simulink model "Q2_Simulink_Model"  (R2018a)
settings: Solver=VariableStepDiscrete  StartTime=0.0  StopTime=4  RelTol=1e-3
libraries: powerlib x22, pePowerMeasurement x4
settings Model: NumberOfSteps=10  Creator=Ataseven  LastModifiedBy=etkiacilan
settings ConfigComp: DVTestSuiteOptimization=CombinedObjectives (Nonlinear Extended)  DVDetectFloatOverflow=off

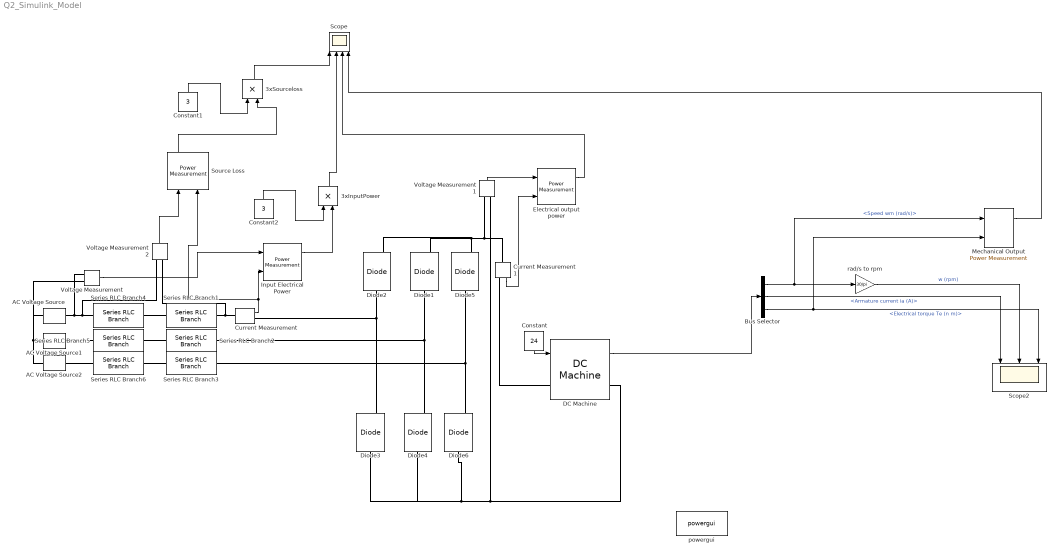
== system Q2_Simulink_Model ==
  3xInputPower : Product
  3xSourceloss : Product
  AC Voltage Source : powerlib/Electrical Sources/AC Voltage Source  Amplitude=326.59863  Phase=0  Frequency=50  SampleTime=0  Measurements=None  BusType=swing  Pref=10e3  Qref=0  Qmin=-inf  Qmax=+inf
  AC Voltage Source1 : powerlib/Electrical Sources/AC Voltage Source  Amplitude=326.59863  Phase=240  Frequency=50  SampleTime=0  Measurements=None  BusType=swing  Pref=10e3  Qref=0  Qmin=-inf  Qmax=+inf
  AC Voltage Source2 : powerlib/Electrical Sources/AC Voltage Source  Amplitude=326.59863  Phase=120  Frequency=50  SampleTime=0  Measurements=None  BusType=swing  Pref=10e3  Qref=0  Qmin=-inf  Qmax=+inf
  Bus Selector : BusSelector  OutputSignals=Speed wm (rad/s),Armature current ia (A),Electrical torque Te (n m)
  Constant : Constant  Value=24
  Constant1 : Constant  Value=3
  Constant2 : Constant  Value=3
  Current Measurement : powerlib/Measurements/Current Measurement  PhasorSimulation=off  OutputType=Complex  PSBequivalent=0
  Current Measurement1 : powerlib/Measurements/Current Measurement  PhasorSimulation=off  OutputType=Complex  PSBequivalent=0
  DC Machine : powerlib/Machines/DC Machine  PresetModel=No  MechanicalLoad=Torque TL  FieldType=Permanent magnet  ShowDetailedParameters=on  MeasurementBus=off  RLa=[ 10 0.01]  RLf="[ 240  120]"  Laf=1.8  MachineConstant=Back-emf constant (V/rpm)  Ke=0.3  Kt=1.8  J=0.4  Bm=0  Tf=0  w0=1  Ifinit=1  TsPowergui=0  TsBlock=-1
  Diode{1..6} (6 alike) : powerlib/Power Electronics/Diode  Ron=0.02  Lon=0  Vf=0.8  IC=0  UseSnubber=0  Rs=500e6  Cs=250e-9  Measurements=on
  "Electrical output power " : pePowerMeasurement/Power Measurement  OverrideUsingVariant=Discrete  F=50  K=[0 1 2 3]  Ts=10e-6
  Input Electrical Power : pePowerMeasurement/Power Measurement  OverrideUsingVariant=Discrete  F=50  K=[0 1 2 3]  Ts=10e-6
  "Mechanical Output " : pePowerMeasurement/Power Measurement  OverrideUsingVariant=Discrete  F=50  K=[0 1 2 3]  Ts=10e-6
  Scope : Scope  NumInputPorts=4
  Scope2 : Scope  NumInputPorts=3
  Series RLC Branch1 : powerlib/Elements/Series RLC Branch  LConnTagsString=__new0  RConnTagsString=__new0  BranchType=L  Resistance=1  Inductance=100e-6  SetiL0=off  InitialCurrent=0  Capacitance=1e-6  Setx0=off  InitialVoltage=0  Measurements=None
  Series RLC Branch2 : powerlib/Elements/Series RLC Branch  LConnTagsString=__new0  RConnTagsString=__new0  BranchType=L  Resistance=1  Inductance=100e-6  SetiL0=off  InitialCurrent=0  Capacitance=1e-6  Setx0=off  InitialVoltage=0  Measurements=None
  Series RLC Branch3 : powerlib/Elements/Series RLC Branch  LConnTagsString=__new0  RConnTagsString=__new0  BranchType=L  Resistance=1  Inductance=100e-6  SetiL0=off  InitialCurrent=0  Capacitance=1e-6  Setx0=off  InitialVoltage=0  Measurements=None
  Series RLC Branch4 : powerlib/Elements/Series RLC Branch  LConnTagsString=__new0  RConnTagsString=__new0  BranchType=R  Resistance=0.1  Inductance=1e-3  SetiL0=off  InitialCurrent=0  Capacitance=1e-6  Setx0=off  InitialVoltage=0  Measurements=None
  Series RLC Branch5 : powerlib/Elements/Series RLC Branch  LConnTagsString=__new0  RConnTagsString=__new0  BranchType=R  Resistance=0.1  Inductance=1e-3  SetiL0=off  InitialCurrent=0  Capacitance=1e-6  Setx0=off  InitialVoltage=0  Measurements=None
  Series RLC Branch6 : powerlib/Elements/Series RLC Branch  LConnTagsString=__new0  RConnTagsString=__new0  BranchType=R  Resistance=0.1  Inductance=1e-3  SetiL0=off  InitialCurrent=0  Capacitance=1e-6  Setx0=off  InitialVoltage=0  Measurements=None
  "Source Loss " : pePowerMeasurement/Power Measurement  OverrideUsingVariant=Discrete  F=50  K=[0 1 2 3]  Ts=10e-6
  Voltage Measurement : powerlib/Measurements/Voltage Measurement  PhasorSimulation=off  OutputType=Complex  PSBequivalent=0
  Voltage Measurement1 : powerlib/Measurements/Voltage Measurement  PhasorSimulation=off  OutputType=Complex  PSBequivalent=0
  Voltage Measurement2 : powerlib/Measurements/Voltage Measurement  PhasorSimulation=off  OutputType=Complex  PSBequivalent=0
  powergui : powerlib/powergui  Priority=1  SimulationMode=Discrete  SampleTime=10e-6  frequency=60  Iterations=50  frequencyindice=50  Pbase=100e6  ErrMax=1e-4  UnitsV=kV  UnitsW=MW  buscounter=0  FunctionMessages=off  echomessages=off  EnableUseOfTLC=off  CurrentSourceSwitches=off  DisableSnubberDevices=off  DisableRonSwitches=off  DisableVfSwitches=off  DisplayEquations=off  SolverType=Tustin/Backward Euler (TBE)  Interpol=off  ExternalGateDelay=off  methode=off  Ts=100  x0status=blocks  SPID=on  SwTol=0  HookPort=off  RestoreLinks=warning  ResistiveCurrentMeasurement=off  Frange=[0:2:500]  Ylog=off  Xlog=on  ShowGrid=off  save=off  variable=ZData  structure=ScopeData  ZoomFFT=on  StartTime=3  cycles=10  DisplayStyle=1  fundamental=50  FreqAxis=on  MaxFrequency=1000  frequencyindicesteady=1  RmsSteady=1  display=off
  rad/s to rpm : Gain  Gain=30/pi
  wires:
  Bus Selector/1 -> rad/s to rpm/1, "Mechanical Output "/1  "<Speed wm (rad/s)>"
  DC Machine/1 -> Bus Selector/1
  Bus Selector/2 -> Scope2/1  "<Armature current ia (A)>"
  rad/s to rpm/1 -> Scope2/2  "w (rpm)"
  Constant/1 -> DC Machine/1
  Bus Selector/3 -> Scope2/3, "Mechanical Output "/2  "<Electrical torque Te (n m)>"
  "Mechanical Output "/1 -> Scope/4
  Voltage Measurement/1 -> Input Electrical Power/1
  Current Measurement/1 -> "Source Loss "/2, Input Electrical Power/2
  Voltage Measurement1/1 -> "Electrical output power "/1
  Voltage Measurement2/1 -> "Source Loss "/1
  "Source Loss "/1 -> 3xSourceloss/2
  "Electrical output power "/1 -> Scope/3
  Current Measurement1/1 -> "Electrical output power "/2
  Constant1/1 -> 3xSourceloss/1
  3xSourceloss/1 -> Scope/1
  Constant2/1 -> 3xInputPower/1
  3xInputPower/1 -> Scope/2
  Input Electrical Power/1 -> 3xInputPower/2
  connections:
  Series RLC Branch4/LConn1 -- Series RLC Branch1/RConn1
  Diode4/RConn1 -- Series RLC Branch2/LConn1 -- Diode1/LConn1
  Diode6/RConn1 -- Diode5/LConn1 -- Series RLC Branch3/LConn1
  Series RLC Branch5/RConn1 -- AC Voltage Source1/RConn1
  Diode3/RConn1 -- Current Measurement/RConn1 -- Diode2/LConn1
  Series RLC Branch6/LConn1 -- Series RLC Branch3/RConn1
  Series RLC Branch2/RConn1 -- Series RLC Branch5/LConn1
  Series RLC Branch6/RConn1 -- AC Voltage Source2/RConn1
  Diode2/RConn1 -- Diode1/RConn1 -- Diode5/RConn1 -- Current Measurement1/LConn1 -- Voltage Measurement1/LConn1
  Series RLC Branch4/RConn1 -- Voltage Measurement2/LConn1 -- Voltage Measurement/LConn1 -- AC Voltage Source/RConn1
  AC Voltage Source2/LConn1 -- Voltage Measurement/LConn2 -- AC Voltage Source/LConn1 -- AC Voltage Source1/LConn1
  Current Measurement/LConn1 -- Voltage Measurement2/LConn2 -- Series RLC Branch1/LConn1
  Diode6/LConn1 -- Diode4/LConn1 -- Diode3/LConn1 -- Voltage Measurement1/LConn2 -- DC Machine/RConn1
  Current Measurement1/RConn1 -- DC Machine/LConn1
